simulink model "tricycle_TargetpoinT"  (R2021a)
settings: Solver=VariableStepAuto  StartTime=0.0  StopTime=inf  RelTol=1e-3
libraries: simulink_extras x3, vehdynlibviscommon x1
settings Model: Creator=EGYPT  LastModifiedBy=Mostafa Ali
settings SolverCC: AlgebraicLoopSolver=TrustRegion
settings DebuggingCC: SFMachineParentedDataDiag=warning

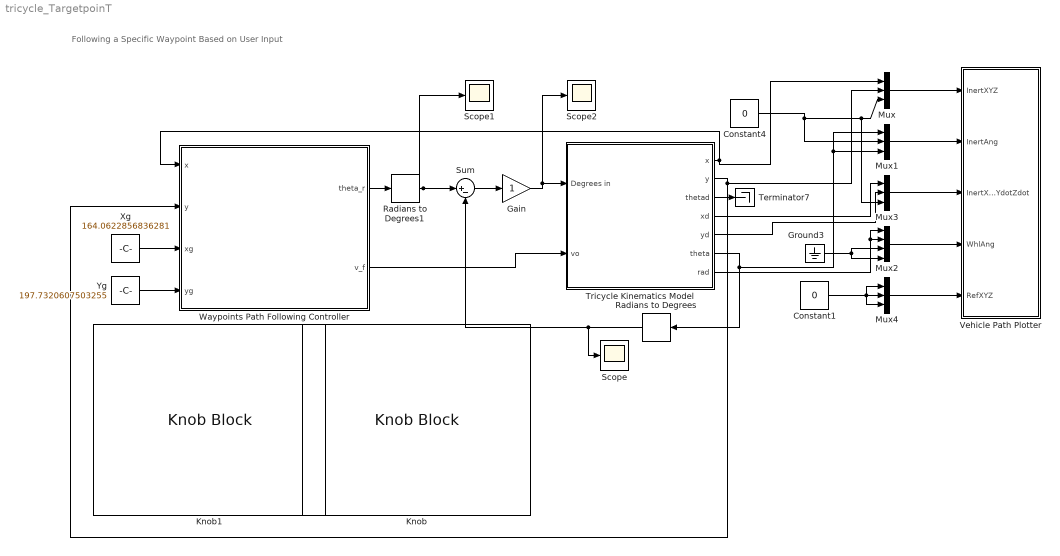
== system tricycle_TargetpoinT ==
  note: Following a Specific Waypoint Based on User Input
  " Tricycle Kinematics Model " : Subsystem
      mask Display: image('D:\grad 1\matlab\maskKM.JPG'); % Use "Edit Image" on toolstrip to change.
  Constant1 : Constant  Value=0
  Constant4 : Constant  Value=0
  Gain : Gain
  Ground3 : Ground
  Knob : KnobBlock  ScaleMax=250
  Knob1 : KnobBlock  ScaleMax=250
  Mux{,1,3..4} (4 alike) : Mux  Inputs=3
  Mux2 : Mux
  Radians to Degrees : simulink_extras/Transformations/Radians to Degrees
  Radians to Degrees1 : simulink_extras/Transformations/Radians to Degrees
  Scope : Scope
  Scope1 : Scope
  Scope2 : Scope
  Sum : Sum  Inputs=|+-
  Terminator7 : Terminator
  Vehicle Path Plotter : Subsystem  mask(Vehicle XY Plotter){extRef=on, extStats=off, extTireF=off, a=2, b=2, w=2, figBorder=10, bufferSize=1024, velNorm=5, tireFNorm=1000, pltDT=0.2}
      mask prompts: extRef "Plot path reference, extRef"; extStats "Display speed, RPM and Gear"; extTireF "Display tire forces"; a "Distance to front axle from CG, a [m]:"; b "Distance to rear axle from CG, b [m]:"; w "Track width, w [m]:"; figBorder "Distance to figure borders, figBorder [m]:"; bufferSize "Path buffer sampe size, bufferSize []:"; velNorm "Velocity vector scaling, velNorm [m*s/m]:"; tireFNorm "Tire force vector scaling, tireFNorm [m/N]:"; pltDT "Plot update rate, pltDT [s]:"
      mask help:
      | This block will display a MATLAB figure which indicates the vehicle path, current position and heading velocity.
      | An optional path reference is also provided.
      mask init:
      | block = gcb;
      | if autoblkschecksimstopped(block)
      |     ParamNames = {'extRef';'extStats';'extTireF';'extTireF'};
      |     PortNames = {'RefXYZ';'Stats';'TireFx';'TireFy'};
      |     for idx=1:length(PortNames)
      |         InportOption  = {'built-in/Ground', [PortNames{idx}, ' Ground'];...
      |             'built-in/Inport',PortNames{idx}};
      |         if ~strcmp(get_param(block,ParamNames{idx}),'on')
      |             NewBlkHdl = autoblksreplaceblock(block, InportOption, 1);
      |             set_param(NewBlkHdl, 'ShowName', 'off');
      |         else
      |             autoblksreplaceblock(block, InportOption, 2);
      |         end
      |     end
      |     InportNames = {'InertXYZ';'InertAng';'InertXdotYdotZdot';'WhlAng';'RefXYZ';'Stats';'TireFx';'TireFy'};
      |     FoundNames = get_param(find_system(block, 'LookUnderMasks', 'all', 'SearchDepth', 1, 'FollowLinks', 'on', 'BlockType', 'Inport'), 'Name');
      |     [~,PortI] = intersect(InportNames, FoundNames);
      |     PortI = sort(PortI);
      |     for idx = 1:length(PortI)
      |         set_param([block, '/', InportNames{PortI(idx)}], 'Port', num2str(idx));
      |     end
      | end
      mask TypeOptions a: Vehicle XY Plotter/a
      mask TypeOptions b: Vehicle XY Plotter/b
      mask TypeOptions w: Vehicle XY Plotter/w
      mask TypeOptions figBorder: Vehicle XY Plotter/figBorder
      mask TypeOptions bufferSize: Vehicle XY Plotter/bufferSize
      mask TypeOptions velNorm: Vehicle XY Plotter/velNorm
      mask TypeOptions tireFNorm: Vehicle XY Plotter/tireFNorm
      mask DialogControl Container3 Prompt: Plot and Display Options
  "Waypoints Path Following Controller " : MATLAB Function  TreatAsAtomicUnit=on
  Xg : Constant  Value=164.0622856836281
  Yg : Constant  Value=197.7320607503255
  wires:
  " Tricycle Kinematics Model "/4(xd) -> Mux3/1
  Yg/1 -> "Waypoints Path Following Controller "/4(yg)
  Constant4/1 -> Mux1/2, Mux/3, Mux3/3
  Ground3/1 -> Mux2/3, Mux2/4
  Radians to Degrees/1 -> Sum/2, Scope/1
  " Tricycle Kinematics Model "/7(rad) -> Mux2/1, Mux2/2
  "Waypoints Path Following Controller "/1(theta_r) -> Radians to Degrees1/1
  Mux2/1 -> Vehicle Path Plotter/4(WhlAng)
  " Tricycle Kinematics Model "/1(x) -> Mux/1, "Waypoints Path Following Controller "/1(x)
  Mux4/1 -> Vehicle Path Plotter/5(RefXYZ)
  Mux1/1 -> Vehicle Path Plotter/2(InertAng)
  Mux/1 -> Vehicle Path Plotter/1(InertXYZ)
  " Tricycle Kinematics Model "/6(theta) -> Mux1/1, Mux1/3, Radians to Degrees/1
  " Tricycle Kinematics Model "/2(y) -> Mux/2, "Waypoints Path Following Controller "/2(y)
  Mux3/1 -> Vehicle Path Plotter/3(InertXdotYdotZdot)
  " Tricycle Kinematics Model "/5(yd) -> Mux3/2
  Xg/1 -> "Waypoints Path Following Controller "/3(xg)
  Constant1/1 -> Mux4/3, Mux4/1, Mux4/2
  "Waypoints Path Following Controller "/2(v_f) -> " Tricycle Kinematics Model "/2(vo)
  " Tricycle Kinematics Model "/3(thetad) -> Terminator7/1
  Gain/1 -> " Tricycle Kinematics Model "/1(Degrees in), Scope2/1
  Sum/1 -> Gain/1
  Radians to Degrees1/1 -> Scope1/1, Sum/1

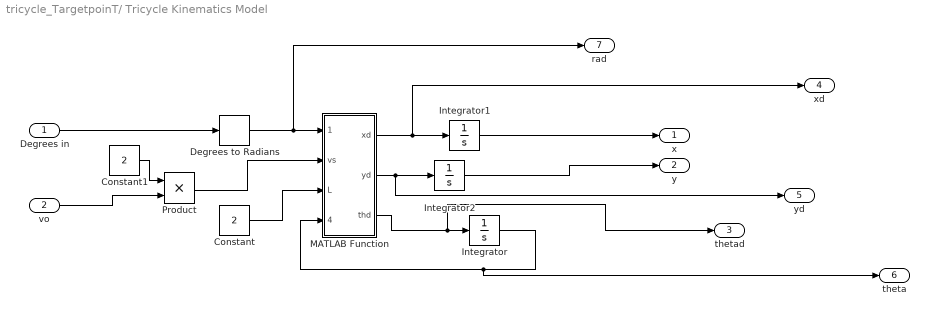
== system tricycle_TargetpoinT/ Tricycle Kinematics Model  ==
  Degrees in : Inport
  vo : Inport  Port=2
  Constant : Constant  Value=2
  Constant1 : Constant  Value=2
  Degrees to Radians : simulink_extras/Transformations/Degrees to Radians
  Integrator : Integrator
  Integrator1 : Integrator
  Integrator2 : Integrator
  MATLAB Function : MATLAB Function  TreatAsAtomicUnit=on
  Product : Product
  x : Outport
  y : Outport  Port=2
  thetad : Outport  Port=3
  xd : Outport  Port=4
  yd : Outport  Port=5
  theta : Outport  Port=6
  rad : Outport  Port=7
  wires:
  Integrator/1 -> theta/1, MATLAB Function/4(theta_r)
  Degrees to Radians/1 -> rad/1, MATLAB Function/1(delta_r)
  MATLAB Function/1(xd) -> xd/1, Integrator1/1
  Integrator2/1 -> y/1
  Product/1 -> MATLAB Function/2(vs)
  MATLAB Function/3(thd) -> thetad/1, Integrator/1
  Constant/1 -> MATLAB Function/3(L)
  MATLAB Function/2(yd) -> yd/1, Integrator2/1
  Constant1/1 -> Product/1
  Degrees in/1 -> Degrees to Radians/1
  Integrator1/1 -> x/1
  vo/1 -> Product/2

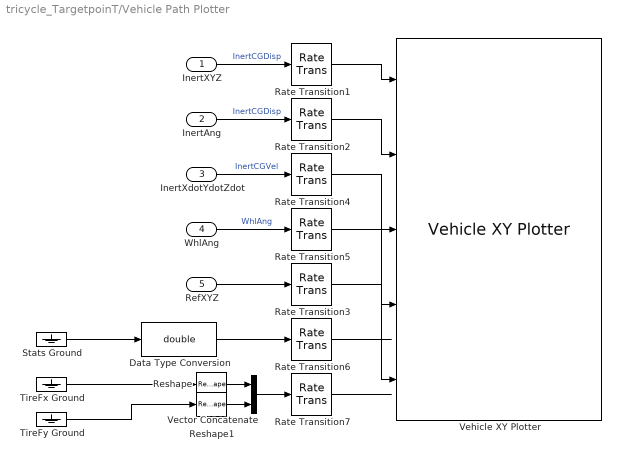
== system tricycle_TargetpoinT/Vehicle Path Plotter ==
  InertXYZ : Inport
  InertAng : Inport  Port=2
  InertXdotYdotZdot : Inport  Port=3
  WhlAng : Inport  Port=4
  RefXYZ : Inport  Port=5
  Data Type Conversion : DataTypeConversion  OutDataTypeStr=double
  Rate Transition{1..7} (7 alike) : RateTransition  Deterministic=off  OutPortSampleTime=pltDT
  Reshape : Reshape  OutputDimensionality=Row vector (2-D)
  Reshape1 : Reshape  OutputDimensionality=Row vector (2-D)
  Stats Ground : Ground
  TireFx Ground : Ground
  TireFy Ground : Ground
  Vector Concatenate : Concatenate  Mode=Multidimensional array
  Vehicle XY Plotter : vehdynlibviscommon/Vehicle XY Plotter  w=w  a=a  b=b  figBorder=figBorder  bufferSize=bufferSize  extStats=off  extTireF=off
      settings: SourceProductBaseCode=VE
  wires:
  Vector Concatenate/1 -> Rate Transition7/1
  Reshape1/1 -> Vector Concatenate/2
  Reshape/1 -> Vector Concatenate/1
  RefXYZ/1 -> Rate Transition3/1
  Rate Transition7/1 -> ?
  Data Type Conversion/1 -> Rate Transition6/1
  Rate Transition6/1 -> ?
  Rate Transition5/1 -> Vehicle XY Plotter/4
  Rate Transition4/1 -> Vehicle XY Plotter/3
  Rate Transition2/1 -> Vehicle XY Plotter/2
  Rate Transition1/1 -> Vehicle XY Plotter/1
  Rate Transition3/1 -> Vehicle XY Plotter/5
  WhlAng/1 -> Rate Transition5/1  "WhlAng"
  InertXYZ/1 -> Rate Transition1/1  "InertCGDisp"
  InertXdotYdotZdot/1 -> Rate Transition4/1  "InertCGVel"
  InertAng/1 -> Rate Transition2/1  "InertCGDisp"
  Stats Ground/1 -> Data Type Conversion/1
  TireFx Ground/1 -> Reshape/1
  TireFy Ground/1 -> Reshape1/1

== matlab function tricycle_TargetpoinT/Waypoints Path Following Controller  ==
  data: x input; y input; theta_r output; xg input; yg input; v_f output
function [theta_r,v_f]   = fcn(x,y,xg,yg)
v_f=0
dx=xg-x
dy=yg-y
q=((dx)^2)+((dy)^2)
r=sqrt(q)
theta_r=atan2(dy,dx)
pause(0.001);

if (r>0&&r<1)
     v_f=0;
     
 elseif (r>1)
     v_f=1;
else 
    v_f=0;
end

== matlab function tricycle_TargetpoinT/ Tricycle Kinematics Model /MATLAB Function ==
  data: delta_r input; xd output; yd output; thd output; vs input; L input; theta_r input
function[xd,yd,thd] = fcn(delta_r,vs,L,theta_r)
xd=vs*cos(delta_r)*cos(theta_r)
yd=vs*cos(delta_r)*sin(theta_r)
thd=(vs/L)*sin(delta_r)
